simulink model "PWMSubsystem"  (R2017a)
settings: Solver=VariableStepAuto  StartTime=0.0  StopTime=10.0  RelTol=1e-3
settings Model: Creator=Rutvik  LastModifiedBy=Rutvik

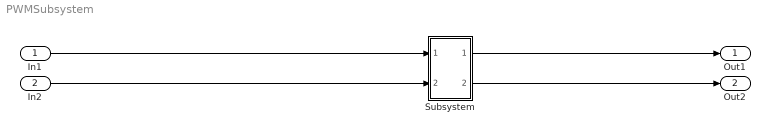
== system PWMSubsystem ==
  In1 : Inport
  In2 : Inport  Port=2
  Subsystem : Subsystem
  Out1 : Outport
  Out2 : Outport  Port=2
  wires:
  In1/1 -> Subsystem/1(In1)
  In2/1 -> Subsystem/2(In2)
  Subsystem/1(Out1) -> Out1/1
  Subsystem/2(Out2) -> Out2/1

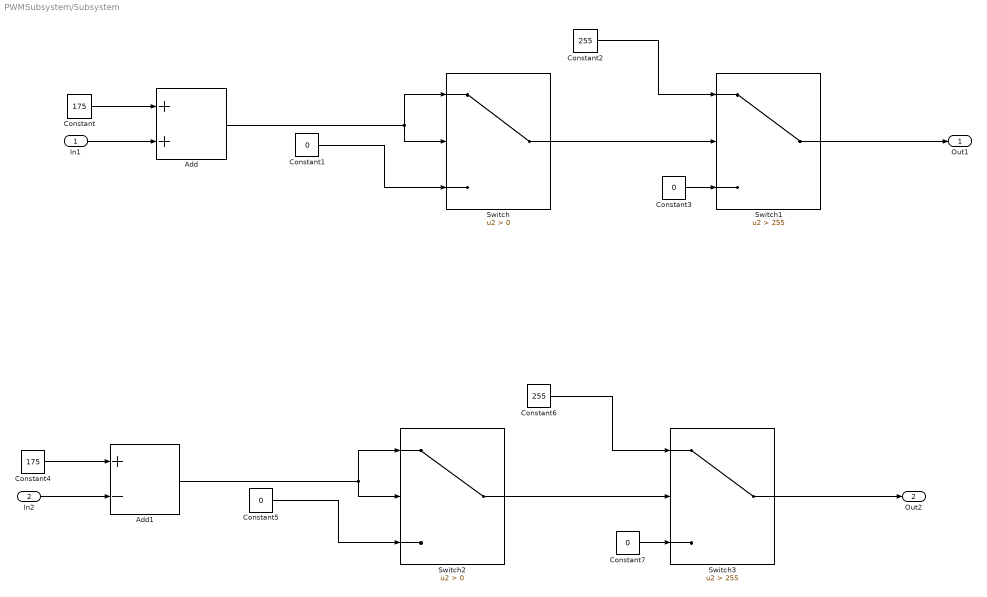
== system PWMSubsystem/Subsystem ==
  In1 : Inport
  In2 : Inport  Port=2
  Add : Sum
  Add1 : Sum  Inputs=+-
  Constant : Constant  Value=175
  Constant{1,3,5,7} (4 alike) : Constant  Value=0
  Constant2 : Constant  Value=255
  Constant4 : Constant  Value=175
  Constant6 : Constant  Value=255
  Switch : Switch  Criteria=u2 > Threshold
  Switch1 : Switch  Criteria=u2 > Threshold  Threshold=255
  Switch2 : Switch  Criteria=u2 > Threshold
  Switch3 : Switch  Criteria=u2 > Threshold  Threshold=255
  Out1 : Outport
  Out2 : Outport  Port=2
  wires:
  In1/1 -> Add/2
  Constant/1 -> Add/1
  Constant2/1 -> Switch1/1
  Switch1/1 -> Out1/1
  Add/1 -> Switch/1, Switch/2
  Switch/1 -> Switch1/2
  Constant6/1 -> Switch3/1
  Switch2/1 -> Switch3/2
  Add1/1 -> Switch2/1, Switch2/2
  In2/1 -> Add1/2
  Constant7/1 -> Switch3/3
  Constant5/1 -> Switch2/3
  Switch3/1 -> Out2/1
  Constant4/1 -> Add1/1
  Constant3/1 -> Switch1/3
  Constant1/1 -> Switch/3
